simulink model "H6_Truck_System"  (R2026a)
settings: Solver=ode45  StopTime=120  MaxStep=0.05  RelTol=1e-4  AbsTol=1e-5
libraries: slpidlib x1
settings Model: Creator=RICARDO  LastModifiedBy=RICARDO

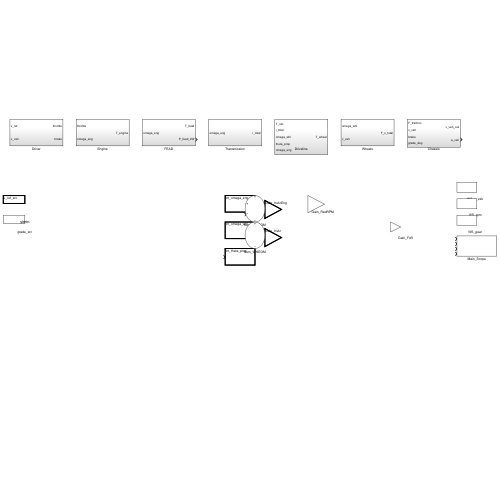
[thumbnail: Simulink's stored preview of the top-level diagram]
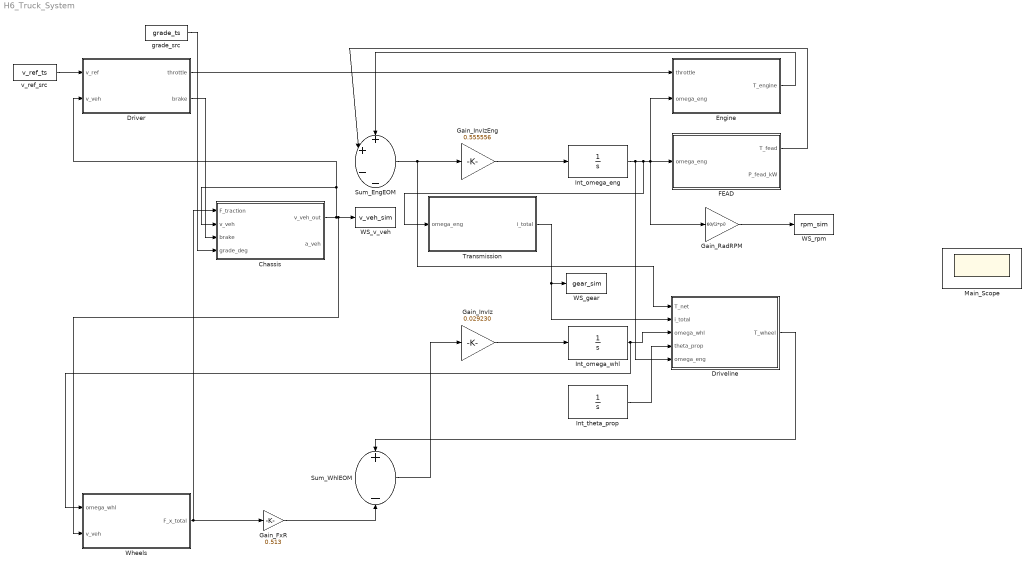
== system H6_Truck_System ==
  Chassis : Subsystem
  Driveline : Subsystem
  Driver : Subsystem
  Engine : Subsystem
  FEAD : Subsystem
  Gain_FxR : Gain  Gain=0.513
  Gain_InvIz : Gain  Gain=0.029230
  Gain_InvIzEng : Gain  Gain=0.555556
  Gain_RadRPM : Gain  Gain=60/(2*pi)
  Int_omega_eng : Integrator  InitialCondition=600*2*pi/60  LowerSaturationLimit=0
  Int_omega_whl : Integrator  LowerSaturationLimit=0
  Int_theta_prop : Integrator
  Main_Scope : Scope  NumInputPorts=4
  Sum_EngEOM : Sum  Inputs=++--
  Sum_WhlEOM : Sum  Inputs=+-
  Transmission : Subsystem
  WS_gear : ToWorkspace  VariableName=gear_sim  SampleTime=-1
  WS_rpm : ToWorkspace  VariableName=rpm_sim  SampleTime=-1
  WS_v_veh : ToWorkspace  VariableName=v_veh_sim  SampleTime=-1
  Wheels : Subsystem
  grade_src : FromWorkspace  VariableName=grade_ts
  v_ref_src : FromWorkspace  VariableName=v_ref_ts
  wires:
  Chassis/1(v_veh_out) -> Wheels/2(v_veh), WS_v_veh/1, Driver/2(v_veh), Chassis/2(v_veh)
  v_ref_src/1 -> Driver/1(v_ref)
  grade_src/1 -> Chassis/4(grade_deg)
  Driver/1(throttle) -> Engine/1(throttle)
  Wheels/1(F_x_total) -> Chassis/1(F_traction), Gain_FxR/1
  Driver/2(brake) -> Chassis/3(brake)
  Gain_FxR/1 -> Sum_WhlEOM/2
  Sum_EngEOM/1 -> Driveline/1(T_net), Gain_InvIzEng/1
  FEAD/1(T_fead) -> Sum_EngEOM/2
  Sum_WhlEOM/1 -> Gain_InvIz/1
  Gain_InvIzEng/1 -> Int_omega_eng/1
  Transmission/1(i_total) -> Driveline/2(i_total), WS_gear/1
  Int_theta_prop/1 -> Driveline/4(theta_prop)
  Gain_InvIz/1 -> Int_omega_whl/1
  Int_omega_eng/1 -> Engine/2(omega_eng), Gain_RadRPM/1, FEAD/1(omega_eng), Transmission/1(omega_eng), Driveline/5(omega_eng)
  Int_omega_whl/1 -> Wheels/1(omega_whl), Driveline/3(omega_whl)
  Engine/1(T_engine) -> Sum_EngEOM/1
  Gain_RadRPM/1 -> WS_rpm/1
  Driveline/1(T_wheel) -> Sum_WhlEOM/1

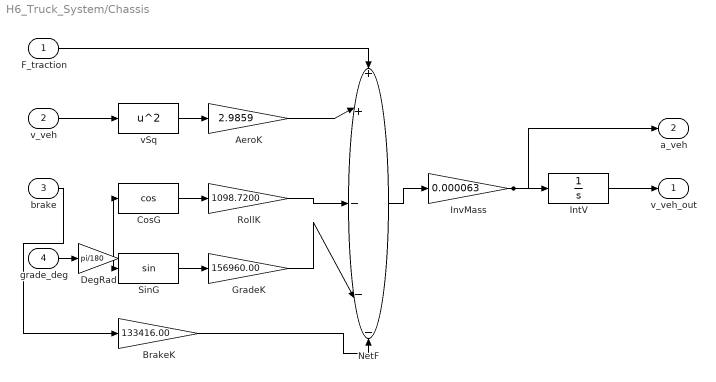
== system H6_Truck_System/Chassis ==
  F_traction : Inport
  v_veh : Inport  Port=2
  brake : Inport  Port=3
  grade_deg : Inport  Port=4
  AeroK : Gain  Gain=2.9859
  BrakeK : Gain  Gain=133416.00
  CosG : Trigonometry  Operator=cos
  DegRad : Gain  Gain=pi/180
  GradeK : Gain  Gain=156960.00
  IntV : Integrator  LowerSaturationLimit=0
  InvMass : Gain  Gain=0.000063
  NetF : Sum  Inputs=++---
  RollK : Gain  Gain=1098.7200
  SinG : Trigonometry
  vSq : Math  Operator=square
  v_veh_out : Outport
  a_veh : Outport  Port=2
  wires:
  grade_deg/1 -> DegRad/1
  DegRad/1 -> CosG/1, SinG/1
  v_veh/1 -> vSq/1
  vSq/1 -> AeroK/1
  CosG/1 -> RollK/1
  SinG/1 -> GradeK/1
  brake/1 -> BrakeK/1
  F_traction/1 -> NetF/1
  AeroK/1 -> NetF/2
  RollK/1 -> NetF/3
  GradeK/1 -> NetF/4
  BrakeK/1 -> NetF/5
  NetF/1 -> InvMass/1
  InvMass/1 -> IntV/1, a_veh/1
  IntV/1 -> v_veh_out/1

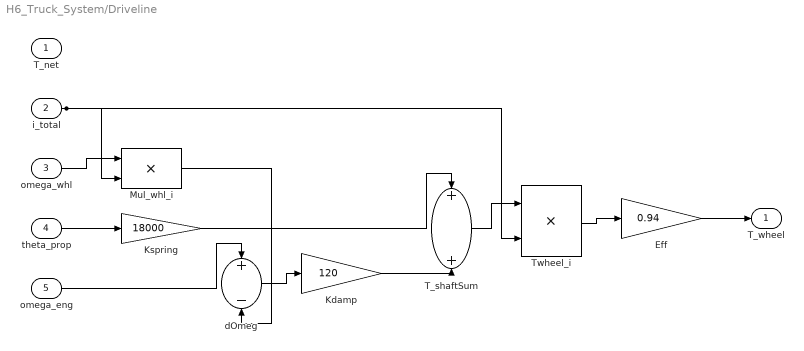
== system H6_Truck_System/Driveline ==
  T_net : Inport
  i_total : Inport  Port=2
  omega_whl : Inport  Port=3
  theta_prop : Inport  Port=4
  omega_eng : Inport  Port=5
  Eff : Gain  Gain=0.94
  Kdamp : Gain  Gain=120
  Kspring : Gain  Gain=18000
  Mul_whl_i : Product
  T_shaftSum : Sum
  Twheel_i : Product
  dOmeg : Sum  Inputs=+-
  T_wheel : Outport
  wires:
  omega_whl/1 -> Mul_whl_i/1
  i_total/1 -> Mul_whl_i/2, Twheel_i/2
  theta_prop/1 -> Kspring/1
  omega_eng/1 -> dOmeg/1
  Mul_whl_i/1 -> dOmeg/2
  dOmeg/1 -> Kdamp/1
  Kspring/1 -> T_shaftSum/1
  Kdamp/1 -> T_shaftSum/2
  T_shaftSum/1 -> Twheel_i/1
  Twheel_i/1 -> Eff/1
  Eff/1 -> T_wheel/1

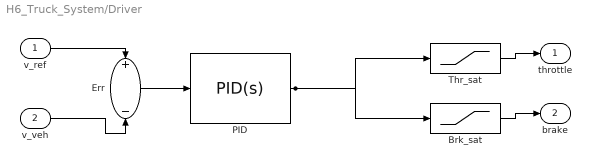
== system H6_Truck_System/Driver ==
  v_ref : Inport
  v_veh : Inport  Port=2
  Brk_sat : Saturate  UpperLimit=1  LowerLimit=0
  Err : Sum  Inputs=+-
  PID : slpidlib/PID Controller  Controller=PID  Form=Parallel  TimeDomain=Continuous-time  UseExternalTs=off  SampleTime=-1  IntegratorMethod=Forward Euler  FilterMethod=Forward Euler  ControllerParametersSource=internal  P=800  I=120  UseKiTs=off  D=30  UseExternalDerivativeSource=off  N=50  UseFilter=on  TunerSelectOption=Transfer Function Based (PID Tuner App)  InitialConditionSource=internal  InitialConditionForIntegrator=0  InitialConditionForFilter=0  DifferentiatorICPrevScaledInput=0  ExternalReset=none  TrackingMode=off  Kt=1  LimitOutput=off  SatLimitsSource=internal  UpperSaturationLimit=inf  LowerSaturationLimit=-inf  LinearizeAsGain=on  AntiWindupMode=none  Kb=1  LimitIntegrator=off  UpperIntegratorSaturationLimit=inf  LowerIntegratorSaturationLimit=-inf  POutMin=[]  POutMax=[]  IOutMin=[]  IOutMax=[]  DOutMin=[]  DOutMax=[]  NOutMin=[]  NOutMax=[]  SumOutMin=[]  SumOutMax=[]  SaturationOutMin=[]  SaturationOutMax=[]  PParamMin=[]  PParamMax=[]  IParamMin=[]  IParamMax=[]  DParamMin=[]  DParamMax=[]  NParamMin=[]  NParamMax=[]  KbParamMin=[]  KbParamMax=[]  KtParamMin=[]  KtParamMax=[]  KbOutMin=[]  KbOutMax=[]  KtOutMin=[]  KtOutMax=[]  IntegratorOutMin=[]  IntegratorOutMax=[]  FilterOutMin=[]  FilterOutMax=[]  SumI1OutMin=[]  SumI1OutMax=[]  SumI2OutMin=[]  SumI2OutMax=[]  SumI3OutMin=[]  SumI3OutMax=[]  SumI4OutMin=[]  SumI4OutMax=[]  SumDOutMin=[]  SumDOutMax=[]  DifferentiatorOutMin=[]  DifferentiatorOutMax=[]  FilterDiffOutCoefMin=[]  FilterDiffOutCoefMax=[]  ReciprocalOutMin=[]  ReciprocalOutMax=[]  SumDenOutMin=[]  SumDenOutMax=[]  SumNumOutMin=[]  SumNumOutMax=[]  DivideOutMin=[]  DivideOutMax=[]  UdiffTsProdOutMin=[]  UdiffTsProdOutMax=[]  NTsProdOutMin=[]  NTsProdOutMax=[]  UintegralTsProdOutMin=[]  UintegralTsProdOutMax=[]  UngainTsProdOutMin=[]  UngainTsProdOutMax=[]  ClampingZeroOutDataTypeStr=Inherit: Inherit via back propagation  ClampingZeroOutMin=[]  ClampingZeroOutMax=[]  FilterDenConstantOutDataTypeStr=Inherit: Inherit via back propagation  FilterDenConstantOutMin=[]  FilterDenConstantOutMax=[]  PCopyOutDataTypeStr=Inherit: Inherit via back propagation  PCopyOutMin=[]  PCopyOutMax=[]  NCopyOutDataTypeStr=Inherit: Inherit via back propagation  NCopyOutMin=[]  NCopyOutMax=[]  IntegratorContinuousStateAttributes=''  IntegratorStateMustResolveToSignalObject=off  IntegratorRTWStateStorageClass=Auto  FilterContinuousStateAttributes=''  FilterStateMustResolveToSignalObject=off  FilterRTWStateStorageClass=Auto  ParallelPVariant=InternalParameters  IdealPVariant=Disabled  IVariant=InternalParameters  DVariant=InternalParameters  IntegratorVariant=Continuous  SatVariant=Disabled  AWVariant=Passthrough  PCopyVariant=Disabled  TRVariant=Disabled  FdbkBlocksVariant=Forward  IdealPFdbkVariant=Disabled  SatFdbkVariant=Disabled  DerivativeFilterVariant=ContFilter  NVariant=InternalParameters  NCopyVariant=Disabled  FilterICVariant=InternalICsFilter  IntegratorICVariant=InternalICs  ExternalResetVariant=Disabled  TRSumVariant=Passthrough  SumFdbkVariant=Disabled  SumVariant=Sum_PID  TsampFilterVariant=InternalTs  TsampNgainVariant=Passthrough  TsampIntegralVariant=Disabled_SignalSpec  ExternalSaturationOutDataTypeStr=Inherit: Same as second input  DerivativeSourceVariant=ErrorSignal  PreIntVariant=InternalPreInt
  Thr_sat : Saturate  UpperLimit=1  LowerLimit=0
  throttle : Outport
  brake : Outport  Port=2
  wires:
  v_ref/1 -> Err/1
  v_veh/1 -> Err/2
  Err/1 -> PID/1
  PID/1 -> Thr_sat/1, Brk_sat/1
  Thr_sat/1 -> throttle/1
  Brk_sat/1 -> brake/1

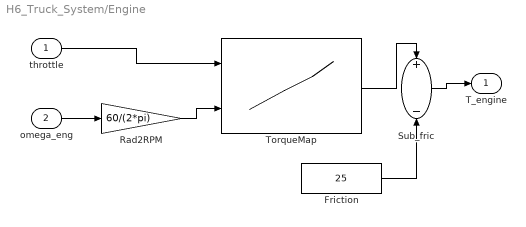
== system H6_Truck_System/Engine ==
  throttle : Inport
  omega_eng : Inport  Port=2
  Friction : Constant  Value=25
  Rad2RPM : Gain  Gain=60/(2*pi)
  Sub_fric : Sum  Inputs=+-
  TorqueMap : Lookup_n-D  BreakpointsForDimension1=[0 0.25 0.5 0.75 1]  BreakpointsForDimension2=[600 800 1000 1200 1400 1600 1800 2000 2200 2400 2500]  Table=[0 0 0 0 0 0 0 0 0 0 0;120 150 175 200 210 210 200 185 165 140 120;240 300 360 420 440 440 420 390 350 300 260;360 500 580 650 680 680 650 610 560 490 420;460 580 680 780 800 800 780 730 680 600 520]  ExtrapMethod=Clip  InternalRulePriority=Speed  RndMeth=Simplest
      settings: InputPortMap=u0,u1
  T_engine : Outport
  wires:
  throttle/1 -> TorqueMap/1
  omega_eng/1 -> Rad2RPM/1
  Rad2RPM/1 -> TorqueMap/2
  TorqueMap/1 -> Sub_fric/1
  Friction/1 -> Sub_fric/2
  Sub_fric/1 -> T_engine/1

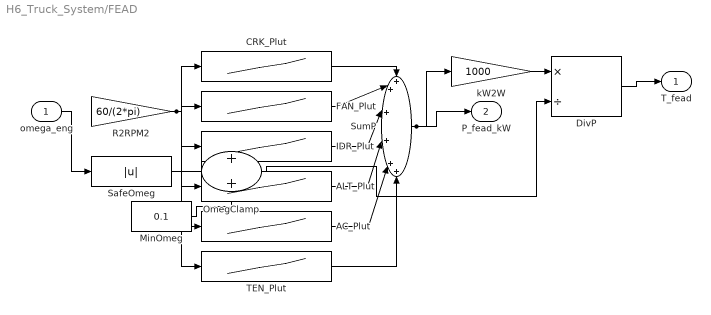
== system H6_Truck_System/FEAD ==
  omega_eng : Inport
  AC_Plut : Lookup_n-D  NumberOfTableDimensions=1  BreakpointsForDimension1=[500 800 1000 1200 1400 1600 1800 2000]  Table=[1 1.33 1.73 2.1 2.42 2.8 3.28 3.64]  ExtrapMethod=Clip  InternalRulePriority=Speed  RndMeth=Simplest
  ALT_Plut : Lookup_n-D  NumberOfTableDimensions=1  BreakpointsForDimension1=[500 800 1000 1200 1400 1600 1800 2000]  Table=[1.6 2.12 2.67 3.06 3.23 3.4 3.55 3.7]  ExtrapMethod=Clip  InternalRulePriority=Speed  RndMeth=Simplest
  CRK_Plut : Lookup_n-D  NumberOfTableDimensions=1  BreakpointsForDimension1=[500 800 1000 1200 1400 1600 1800 2000]  Table=[3.3 4.55 6.54 8.36 10.69 13.2 18.17 22.24]  ExtrapMethod=Clip  InternalRulePriority=Speed  RndMeth=Simplest
  DivP : Product  Inputs=*/
  FAN_Plut : Lookup_n-D  NumberOfTableDimensions=1  BreakpointsForDimension1=[500 800 1000 1200 1400 1600 1800 2000]  Table=[0.5 0.8 1.8 2.8 4.6 6.5 10.8 14.3]  ExtrapMethod=Clip  InternalRulePriority=Speed  RndMeth=Simplest
  IDR_Plut : Lookup_n-D  NumberOfTableDimensions=1  BreakpointsForDimension1=[500 800 1000 1200 1400 1600 1800 2000]  Table=[0.1 0.15 0.17 0.2 0.22 0.25 0.27 0.3]  ExtrapMethod=Clip  InternalRulePriority=Speed  RndMeth=Simplest
  MinOmeg : Constant  Value=0.1
  OmegClamp : Sum
  R2RPM2 : Gain  Gain=60/(2*pi)
  SafeOmeg : Abs  SaturateOnIntegerOverflow=off
  SumP : Sum  Inputs=++++++
  TEN_Plut : Lookup_n-D  NumberOfTableDimensions=1  BreakpointsForDimension1=[500 800 1000 1200 1400 1600 1800 2000]  Table=[0.1 0.15 0.17 0.2 0.22 0.25 0.27 0.27]  ExtrapMethod=Clip  InternalRulePriority=Speed  RndMeth=Simplest
  kW2W : Gain  Gain=1000
  T_fead : Outport
  P_fead_kW : Outport  Port=2
  wires:
  R2RPM2/1 -> CRK_Plut/1, FAN_Plut/1, IDR_Plut/1, ALT_Plut/1, AC_Plut/1, TEN_Plut/1
  CRK_Plut/1 -> SumP/1
  FAN_Plut/1 -> SumP/2
  IDR_Plut/1 -> SumP/3
  ALT_Plut/1 -> SumP/4
  AC_Plut/1 -> SumP/5
  TEN_Plut/1 -> SumP/6
  SumP/1 -> P_fead_kW/1, kW2W/1
  omega_eng/1 -> SafeOmeg/1
  SafeOmeg/1 -> OmegClamp/1
  MinOmeg/1 -> OmegClamp/2
  kW2W/1 -> DivP/1
  OmegClamp/1 -> DivP/2
  DivP/1 -> T_fead/1

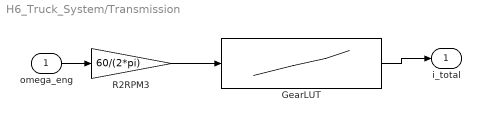
== system H6_Truck_System/Transmission ==
  omega_eng : Inport
  GearLUT : Lookup_n-D  NumberOfTableDimensions=1  BreakpointsForDimension1=[0 850 1100 1350 1650 1950 3000]  Table=[26.896 26.896 15.703 9.717 6.519 4.879 4.1]  ExtrapMethod=Clip  InternalRulePriority=Speed  RndMeth=Simplest
  R2RPM3 : Gain  Gain=60/(2*pi)
  i_total : Outport
  wires:
  omega_eng/1 -> R2RPM3/1
  R2RPM3/1 -> GearLUT/1
  GearLUT/1 -> i_total/1

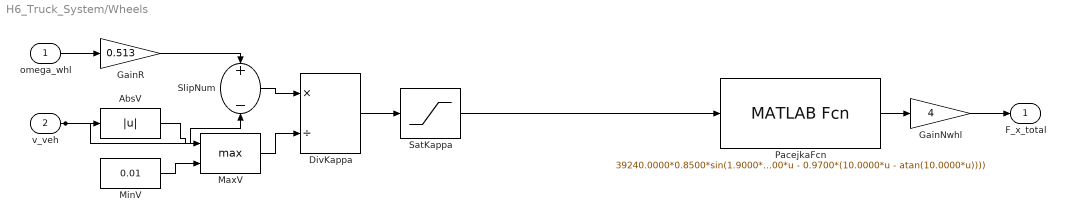
== system H6_Truck_System/Wheels ==
  omega_whl : Inport
  v_veh : Inport  Port=2
  AbsV : Abs  SaturateOnIntegerOverflow=off
  DivKappa : Product  Inputs=*/
  GainNwhl : Gain  Gain=4
  GainR : Gain  Gain=0.513
  MaxV : MinMax  Function=max  Inputs=2
  MinV : Constant  Value=0.01
  PacejkaFcn : MATLABFcn  MATLABFcn=39240.0000*0.8500*sin(1.9000*atan(10.0000*u - 0.9700*(10.0000*u - atan(10.0000*u))))  OutputDimensions=1
  SatKappa : Saturate  UpperLimit=1  LowerLimit=-1
  SlipNum : Sum  Inputs=+-
  F_x_total : Outport
  wires:
  omega_whl/1 -> GainR/1
  GainR/1 -> SlipNum/1
  v_veh/1 -> SlipNum/2, AbsV/1
  AbsV/1 -> MaxV/1
  MinV/1 -> MaxV/2
  SlipNum/1 -> DivKappa/1
  MaxV/1 -> DivKappa/2
  DivKappa/1 -> SatKappa/1
  SatKappa/1 -> PacejkaFcn/1
  PacejkaFcn/1 -> GainNwhl/1
  GainNwhl/1 -> F_x_total/1
